simulink model "elevator_floor"  (R2024b)
settings: Solver=VariableStepAuto  StartTime=0.0  StopTime=inf  RelTol=1e-3
settings Model: Creator=KHALID  LastModifiedBy=DELL

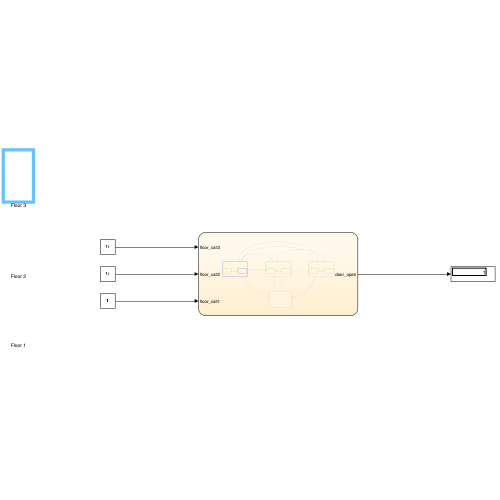
[thumbnail: Simulink's stored preview of the top-level diagram]
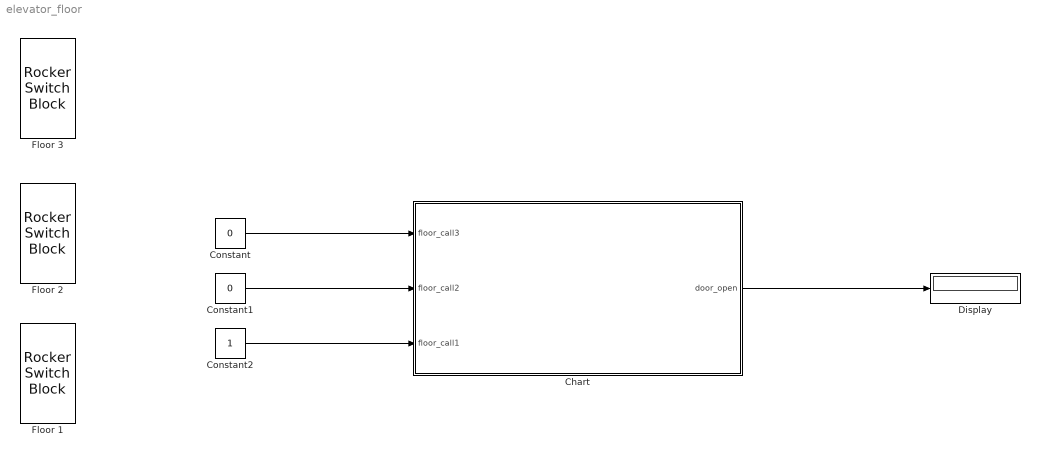
== system elevator_floor ==
  Chart : Stateflow chart  TreatAsAtomicUnit=on
  Constant : Constant  Value=0
  Constant1 : Constant  Value=0
  Constant2 : Constant
  Display : Display
  Floor 1 : RockerSwitchBlock
      settings: Values={{'Off', 'On'}, [0 1]}
  Floor 2 : RockerSwitchBlock
      settings: Values={{'Off', 'On'}, [0 1]}
  Floor 3 : RockerSwitchBlock
      settings: Values={{'Off', 'On'}, [0 1]}
  wires:
  Chart/1(door_open) -> Display/1
  Constant2/1 -> Chart/3(floor_call1)
  Constant1/1 -> Chart/2(floor_call2)
  Constant/1 -> Chart/1(floor_call3)

== stateflow chart elevator_floor/Chart ==
  state Floor_1
    entry:
    disp('Reached First Floor');
    state closed_1
      entry:door_open =0;
      disp('Door Closed');
    state open_1
      entry:door_open =1;
      disp('Door Opened');
    (default) -> closed_1
    open_1 -> closed_1 : [floor_call1==0]
    closed_1 -> open_1 : [floor_call1==1&&floor_call2==0&&floor_call3==0]
  state Floor_2
    entry:
    disp('Reached Second Floor');
    state closed_2
      entry:door_open =0;
      disp('Door Closed');
    state open_2
      entry:door_open =1;
      disp('Door Opened');
    (default) -> closed_2
    open_2 -> closed_2 : [floor_call2==0]
    closed_2 -> open_2 : [floor_call2==1&&floor_call1==0&&floor_call3==0]
  state Floor_3
    entry:
    disp('Reached Third Floor');
    after(5,sec);
    state closed_3
      entry:door_open =0;
      disp('Door Closed');
    state open_3
      entry:door_open =1;
      disp('Door Opened');
    (default) -> closed_3
    open_3 -> closed_3 : [floor_call3==0]
    closed_3 -> open_3 : [floor_call3==1&&floor_call1==0&&floor_call2==0]
  state Elevator_off
    entry:disp('All doors are closed and Elevator is switched off');
  Floor_3 -> Floor_1 [order 1] : [floor_call1==1]
  Floor_1 -> Floor_3 [order 1] : [floor_call3==1&&floor_call1==0&&floor_call2==0]
  Floor_3 -> Floor_2 [order 2] : [floor_call2==1&&floor_call3==0&&floor_call1==0]
  Floor_2 -> Floor_1 [order 2] : [floor_call1==1&&floor_call2==0&&floor_call3==0]
  (default) -> Floor_1
  Floor_1 -> Floor_2 [order 2] : [floor_call1==0&&floor_call3==0]
  Floor_2 -> Floor_3 [order 1] : [floor_call2==0&&floor_call1==0]
  Floor_1 -> Elevator_off [order 3] : [floor_call1==0&&floor_call2==0&&floor_call3==0]{door_open=0}
  Elevator_off -> Floor_1 [order 1] : [floor_call1==1]
  Elevator_off -> Floor_2 [order 2] : [floor_call2==1]
  Floor_2 -> Elevator_off [order 3] : [floor_call1==0&&floor_call2==0&&floor_call3==0]{door_open=0}
  Floor_3 -> Elevator_off [order 3] : [floor_call1==0&&floor_call2==0&&floor_call3==0]{door_open=0}
  Elevator_off -> Floor_3 [order 3] : [floor_call3==1]
  data: floor_call3 input; door_open output; floor_call2 input; floor_call1 input
